simulink model "demo_nv_mano"  (Simulink 6.2)
settings: Solver=ode45  StartTime=0.0  StopTime=200  RelTol=1e-5
libraries: marine_gnc x7, simulink x1
settings Model: LastModifiedBy=perez

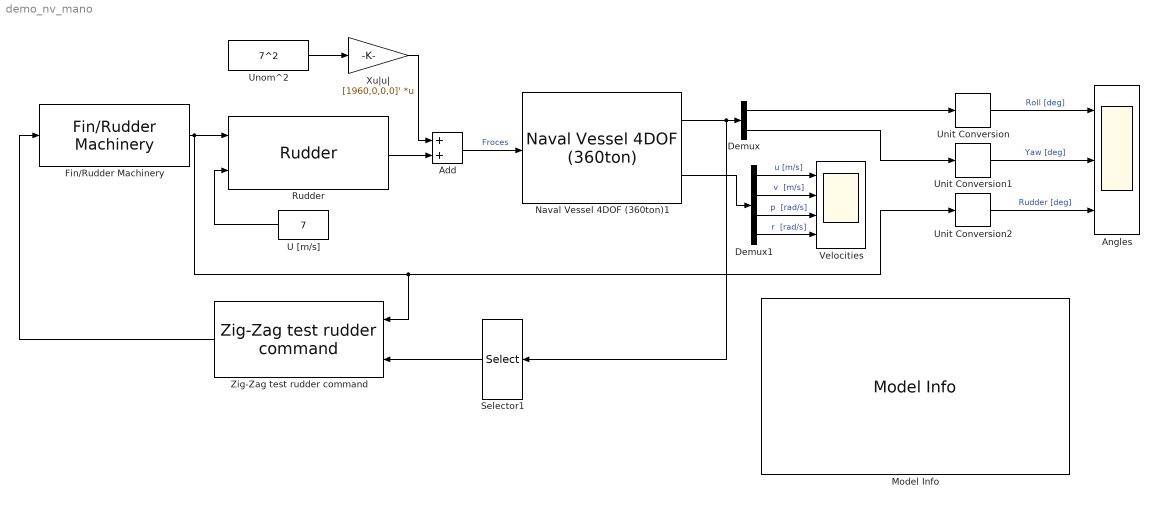
== system demo_nv_mano ==
  Add : Sum  OutScaling=2^-10
  Angles : Scope  NumInputPorts=3
      settings: TimeRange=200  YMin=-10~-100~-50  YMax=10~100~50
  Demux : Demux  Outputs=2
  Demux1 : Demux
  Fin/Rudder Machinery : marine_gnc/Models/Control Surfaces/Fin//Rudder Machinery  Dmax=(pi*45/180)  Dvmax=(pi*20/180)  tc=0.2
  Model Info : simulink/Model-Wide Utilities/Model Info  InitialBlockCM=None  BlockCM=None  Frame=on  DisplayStringWithTags=|  HorizontalTextAlignment=Center  LeftAlignmentValue=0.5  SourceBlockDiagram=demo_nv_mano  TagMaxNumber=20
      | Naval Vessel performing a Zig-Zag Manoeuvre.
      | 
      | Author: Tristan Perez
      | Centre for Ships and Ocean Structures
      | Norwegian University of Science and Technology
      | 
      | Copyright NTNU 2005
      | 
      | Model Created: 2005-04-05
  Naval Vessel 4DOF (360ton)1 : marine_gnc/Examples/Vessels/Naval Vessel 4DOF (360ton)  ic=[7,0,0,0,0,0]'
  Rudder : marine_gnc/Models/Control Surfaces/Rudder  LCG=19.82  VCG=3.36  sp=1.5  ar=3  A=2*1.5  dCL=1.25/(pi*23/180)  CD0=0.0065  stall=(pi*23/180)  rho=1025
  Selector1 : Selector  Orientation=left  Elements=[2]  InputPortWidth=2
  U [m/s] : Constant  Orientation=left  Value=7
  Unit Conversion : marine_gnc/Utilities/Math Operations/Unit Conversion  in=rad2deg
  Unit Conversion1 : marine_gnc/Utilities/Math Operations/Unit Conversion  in=rad2deg
  Unit Conversion2 : marine_gnc/Utilities/Math Operations/Unit Conversion  in=rad2deg
  Unom^2 : Constant  Value=7^2
  Velocities : Scope  NumInputPorts=4
      settings: TimeRange=200  YMin=4~-2~-0.1~-0.1  YMax=8~2~0.1~0.1
  Xu|u| : Gain  Gain=[1960,0,0,0]'  Multiplication=Matrix(K*u)
  "Zig-Zag test rudder command " : marine_gnc/Guidance/Zig-Zag test rudder command   Orientation=left  RL=pi*45/180
  wires:
  Fin/Rudder Machinery/1 -> Rudder/1, "Zig-Zag test rudder command "/1, Unit Conversion2/1
  "Zig-Zag test rudder command "/1 -> Fin/Rudder Machinery/1
  Selector1/1 -> "Zig-Zag test rudder command "/2
  Naval Vessel 4DOF (360ton)1/1 -> Selector1/1, Demux/1
  Add/1 -> Naval Vessel 4DOF (360ton)1/1  "Froces"
  Rudder/1 -> Add/2
  Unom^2/1 -> Xu|u|/1
  Xu|u|/1 -> Add/1
  U [m/s]/1 -> Rudder/2
  Demux1/1 -> Velocities/1  "u [m/s]"
  Naval Vessel 4DOF (360ton)1/2 -> Demux1/1
  Demux1/2 -> Velocities/2  "v  [m/s]"
  Demux1/3 -> Velocities/3  "p  [rad/s]"
  Demux1/4 -> Velocities/4  "r  [rad/s]"
  Unit Conversion/1 -> Angles/1  "Roll [deg]"
  Demux/1 -> Unit Conversion/1
  Unit Conversion1/1 -> Angles/2  "Yaw [deg]"
  Unit Conversion2/1 -> Angles/3  "Rudder [deg]"
  Demux/2 -> Unit Conversion1/1
